simulink model "Cooperative_Localization_05_New2"  (R2016b)
settings: Solver=ode45  StartTime=0.0  StopTime=200  RelTol=1e-3  EnableMultiTasking=on
InitFcn:
  | Const_Coop_Local_05
undefined symbols (not defined in the file): alpha, AN, B, B_pseudo_inverse, BBT_inv, BN, D, Delta_form, Gama0, gamma0, gamma_0, gamma_1, H, K, k0_est, k1, k1_est, k2, KI, Ki_1, Ki_2, Ki_3, Ki_4, lambda, m_cont, Mb, Mu, n, N, n_cont, Observer_Gain, P_struct, Q, Q1, R, Rho1, Rho_0, rho_0, rho_1, t_cont, U_dot0_M
(part 2 of 3)

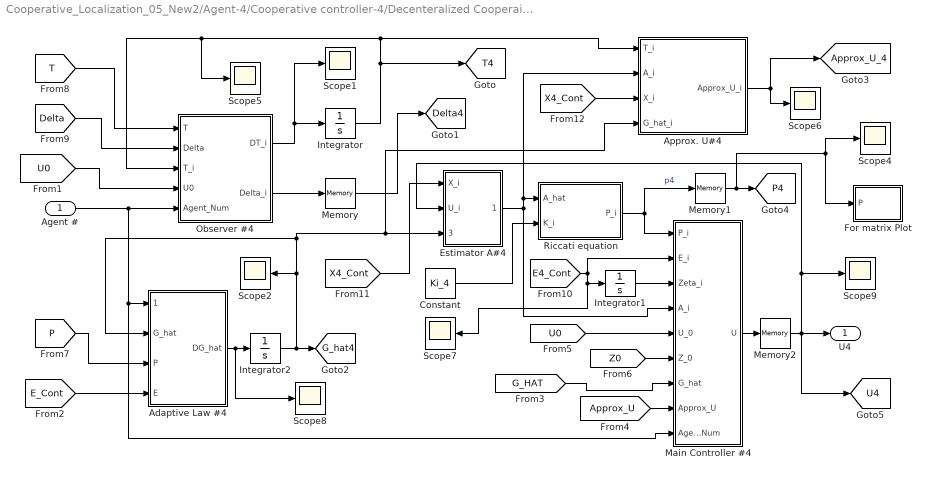
== system Cooperative_Localization_05_New2/Agent-4/Cooperative controller-4/Decenteralized Cooperaive Controller #4 ==
  Agent # : Inport
  Adaptive Law #4 : MATLAB Function  TreatAsAtomicUnit=on
  Approx. U#4 : MATLAB Function  TreatAsAtomicUnit=on
  Constant : Constant  Value=Ki_4
  Estimator A#4 : Subsystem
  For matrix Plot : Subsystem
  Integrator : Integrator  InitialCondition=zeros(n_cont,1)
  Integrator1 : Integrator  InitialCondition=zeros(n_cont,1)
  Integrator2 : Integrator  InitialCondition=zeros(t_cont,1)
  Main Controller #4 : MATLAB Function  TreatAsAtomicUnit=on
  Memory : Memory  X0=zeros(n_cont,1)
  Memory1 : Memory  X0=eye(n_cont)
  Memory2 : Memory  X0=zeros(m_cont,1)
  Observer #4 : MATLAB Function  TreatAsAtomicUnit=on
  Riccati equation : MATLAB Function  TreatAsAtomicUnit=on
  Scope{1..2,4..9} (8 alike) : Scope
  U4 : Outport
  tag scope: Approx_U_4=global, Delta4=global, G_hat4=global, P4=global, T4=global, U4=global
  wires:
  Memory/1 -> [Delta4]
  Agent #/1 -> Main Controller #4/9(Agent_Num), Adaptive Law #4/1(Agent_Num), Observer #4/5(Agent_Num)
  Observer #4/1(DT_i) -> Scope1/1, Integrator/1
  Observer #4/2(Delta_i) -> Memory/1
  [U0] -> Observer #4/4(U0)
  Adaptive Law #4/1(DG_hat) -> Scope8/1, Integrator2/1
  Integrator2/1 -> [G_hat4], Estimator A#4/3(G_hat_i), Approx. U#4/4(G_hat_i), Adaptive Law #4/2(G_hat), Scope2/1
  Integrator/1 -> Approx. U#4/1(T_i), Scope5/1, Observer #4/3(T_i), [T4]
  [Approx_U] -> Main Controller #4/8(Approx_U)
  [G_HAT] -> Main Controller #4/7(G_hat)
  [U0] -> Main Controller #4/5(U_0)
  [Z0] -> Main Controller #4/6(Z_0)
  Estimator A#4/1(A_hat_i) -> Main Controller #4/4(A_i), Riccati equation/1(A_hat), Approx. U#4/2(A_i)
  Riccati equation/1(P_i) -> Main Controller #4/1(P_i), Memory1/1  "p4"
  Main Controller #4/1(U) -> Memory2/1
  [P] -> Adaptive Law #4/3(P)
  [E_Cont] -> Adaptive Law #4/4(E)
  [T] -> Observer #4/1(T)
  [Delta] -> Observer #4/2(Delta)
  [E4_Cont] -> Main Controller #4/2(E_i), Integrator1/1, Scope7/1
  Integrator1/1 -> Main Controller #4/3(Zeta_i)
  [X4_Cont] -> Estimator A#4/1(X_i)
  [X4_Cont] -> Approx. U#4/3(X_i)
  Constant/1 -> Riccati equation/2(K_i)
  Memory2/1 -> [U4], Scope9/1, Estimator A#4/2(U_i), U4/1
  Memory1/1 -> For matrix Plot/1(P), Scope4/1, [P4]
  Approx. U#4/1(Approx_U_i) -> Scope6/1, [Approx_U_4]

== system Cooperative_Localization_05_New2/Agent-4/Relative positions-4/Differentiator_Scalar1 ==
  x_d : Inport
  Integrator : Integrator
  Integrator1 : Integrator
  Memory : Memory
  Scope : Scope
  Scope1 : Scope
  Sliding differentiator : MATLAB Function  TreatAsAtomicUnit=on
  Sliding differentiator1 : MATLAB Function  TreatAsAtomicUnit=on
  Sum : Sum  Inputs=|-+
  Dx_d : Outport
  wires:
  Memory/1 -> Dx_d/1
  Sliding differentiator1/1(Du1) -> Integrator/1
  Integrator/1 -> Sliding differentiator/1(u1)
  x_d/1 -> Sum/1
  Sum/1 -> Scope1/1, Sliding differentiator/2(e_inp), Sliding differentiator1/1(e_inp)
  Integrator1/1 -> Sum/2
  Sliding differentiator/1(u) -> Scope/1, Integrator1/1, Memory/1

== system Cooperative_Localization_05_New2/Agent-4/Relative positions-4/Differentiator_Scalar2 ==
  x_d : Inport
  Integrator : Integrator
  Integrator1 : Integrator
  Memory : Memory
  Scope : Scope
  Scope1 : Scope
  Sliding differentiator : MATLAB Function  TreatAsAtomicUnit=on
  Sliding differentiator1 : MATLAB Function  TreatAsAtomicUnit=on
  Sum : Sum  Inputs=|-+
  Dx_d : Outport
  wires:
  Sliding differentiator/1(u) -> Memory/1, Integrator1/1, Scope/1
  Integrator1/1 -> Sum/2
  Sum/1 -> Sliding differentiator1/1(e_inp), Sliding differentiator/2(e_inp), Scope1/1
  x_d/1 -> Sum/1
  Integrator/1 -> Sliding differentiator/1(u1)
  Sliding differentiator1/1(Du1) -> Integrator/1
  Memory/1 -> Dx_d/1

== system Cooperative_Localization_05_New2/Agent-4/Relative positions-4/Differentiator_Scalar3 ==
  x_d : Inport
  Integrator : Integrator
  Integrator1 : Integrator
  Memory : Memory
  Scope : Scope
  Scope1 : Scope
  Sliding differentiator : MATLAB Function  TreatAsAtomicUnit=on
  Sliding differentiator1 : MATLAB Function  TreatAsAtomicUnit=on
  Sum : Sum  Inputs=|-+
  Dx_d : Outport
  wires:
  Memory/1 -> Dx_d/1
  Sliding differentiator1/1(Du1) -> Integrator/1
  Integrator/1 -> Sliding differentiator/1(u1)
  x_d/1 -> Sum/1
  Sum/1 -> Scope1/1, Sliding differentiator/2(e_inp), Sliding differentiator1/1(e_inp)
  Integrator1/1 -> Sum/2
  Sliding differentiator/1(u) -> Scope/1, Integrator1/1, Memory/1

== system Cooperative_Localization_05_New2/Agent-4/Relative positions-4/Differentiator_Scalar4 ==
  x_d : Inport
  Integrator : Integrator
  Integrator1 : Integrator
  Memory : Memory
  Scope : Scope
  Scope1 : Scope
  Sliding differentiator : MATLAB Function  TreatAsAtomicUnit=on
  Sliding differentiator1 : MATLAB Function  TreatAsAtomicUnit=on
  Sum : Sum  Inputs=|-+
  Dx_d : Outport
  wires:
  Memory/1 -> Dx_d/1
  Sliding differentiator1/1(Du1) -> Integrator/1
  Integrator/1 -> Sliding differentiator/1(u1)
  x_d/1 -> Sum/1
  Sum/1 -> Scope1/1, Sliding differentiator/2(e_inp), Sliding differentiator1/1(e_inp)
  Integrator1/1 -> Sum/2
  Sliding differentiator/1(u) -> Scope/1, Integrator1/1, Memory/1

== system Cooperative_Localization_05_New2/Leader/Ali/Differentiator ==
  x_d : Inport
  Integrator : Integrator  InitialCondition=zeros(n_cont,1)
  Integrator1 : Integrator  InitialCondition=zeros(n_cont,1)
  Scope : Scope
  Scope1 : Scope
  Sliding differentiator : MATLAB Function  TreatAsAtomicUnit=on
  Sliding differentiator1 : MATLAB Function  TreatAsAtomicUnit=on
  Sum : Sum  Inputs=|-+
  Dx_d : Outport
  wires:
  Integrator1/1 -> Sum/2
  Sum/1 -> Sliding differentiator1/1(e), Sliding differentiator/2(e), Scope1/1
  x_d/1 -> Sum/1
  Integrator/1 -> Sliding differentiator/1(u1)
  Sliding differentiator1/1(Du1) -> Integrator/1
  Sliding differentiator/1(u) -> Dx_d/1, Integrator1/1, Scope/1

== system Cooperative_Localization_05_New2/Agent-1/Cooperative controller-1/Decenteralized Cooperaive Controller #1/Estimator A#1 ==
  X_i : Inport
  U_i : Inport  Port=2
  G_hat_i : Inport  Port=3
  Estimation Error : Subsystem
  For matrix Plot1 : Subsystem
  For matrix Plot2 : Subsystem
  Integrator : Integrator  InitialCondition=zeros(n_cont)
  Scope1 : Scope
  Scope5 : Scope
  parameter online identification : MATLAB Function  TreatAsAtomicUnit=on
  A_hat_i : Outport
  tag scope: A_hat1=global
  wires:
  parameter online identification/1(DA_hat) -> For matrix Plot2/1(A_dot), Scope5/1, Integrator/1
  Estimation Error/1(r) -> parameter online identification/1(r)
  Estimation Error/2(wt) -> parameter online identification/2(Wt)
  X_i/1 -> Estimation Error/1(X)
  U_i/1 -> Estimation Error/2(U)
  G_hat_i/1 -> Estimation Error/3(G_hat)
  Integrator/1 -> Scope1/1, For matrix Plot1/1(A), parameter online identification/3(A_hat), [A_hat1], A_hat_i/1

== system Cooperative_Localization_05_New2/Agent-1/Cooperative controller-1/Decenteralized Cooperaive Controller #1/For matrix Plot ==
  P : Inport
  MATLAB Function : MATLAB Function  TreatAsAtomicUnit=on
  To Workspace : ToWorkspace  VariableName=P_1_Cont  SaveFormat=Structure With Time  SampleTime=-1
  wires:
  P/1 -> MATLAB Function/1(u)
  MATLAB Function/1(y) -> To Workspace/1

== system Cooperative_Localization_05_New2/Agent-2/Cooperative controller-2/Decenteralized Cooperaive Controller #2/Estimator A#2 ==
  X_i : Inport
  U_i : Inport  Port=2
  G_hat_i : Inport  Port=3
  Estimation Error : Subsystem
  For matrix Plot1 : Subsystem
  For matrix Plot2 : Subsystem
  Integrator : Integrator  InitialCondition=zeros(n_cont)
  Scope1 : Scope
  Scope5 : Scope
  parameter online identification : MATLAB Function  TreatAsAtomicUnit=on
  A_hat_i : Outport
  tag scope: A_hat2=global
  wires:
  parameter online identification/1(DA_hat) -> For matrix Plot2/1(A_dot), Scope5/1, Integrator/1
  Estimation Error/1(r) -> parameter online identification/1(r)
  Estimation Error/2(wt) -> parameter online identification/2(Wt)
  X_i/1 -> Estimation Error/1(X)
  U_i/1 -> Estimation Error/2(U)
  G_hat_i/1 -> Estimation Error/3(G_hat)
  Integrator/1 -> Scope1/1, For matrix Plot1/1(A), parameter online identification/3(A_hat), [A_hat2], A_hat_i/1

== system Cooperative_Localization_05_New2/Agent-2/Cooperative controller-2/Decenteralized Cooperaive Controller #2/For matrix Plot ==
  P : Inport
  MATLAB Function : MATLAB Function  TreatAsAtomicUnit=on
  To Workspace : ToWorkspace  VariableName=P_2_Cont  SaveFormat=Structure With Time  SampleTime=-1
  wires:
  P/1 -> MATLAB Function/1(u)
  MATLAB Function/1(y) -> To Workspace/1

== system Cooperative_Localization_05_New2/Agent-3/Cooperative controller-3/Decenteralized Cooperaive Controller #3/Estimator A#3 ==
  X_i : Inport
  U_i : Inport  Port=2
  G_hat_i : Inport  Port=3
  Estimation Error : Subsystem
  For matrix Plot1 : Subsystem
  For matrix Plot2 : Subsystem
  Integrator : Integrator  InitialCondition=zeros(n_cont)
  Scope1 : Scope
  Scope5 : Scope
  parameter online identification : MATLAB Function  TreatAsAtomicUnit=on
  A_hat_i : Outport
  tag scope: A_hat3=global
  wires:
  parameter online identification/1(DA_hat) -> For matrix Plot2/1(A_dot), Scope5/1, Integrator/1
  Estimation Error/1(r) -> parameter online identification/1(r)
  Estimation Error/2(wt) -> parameter online identification/2(Wt)
  X_i/1 -> Estimation Error/1(X)
  U_i/1 -> Estimation Error/2(U)
  G_hat_i/1 -> Estimation Error/3(G_hat)
  Integrator/1 -> Scope1/1, For matrix Plot1/1(A), parameter online identification/3(A_hat), [A_hat3], A_hat_i/1

== system Cooperative_Localization_05_New2/Agent-3/Cooperative controller-3/Decenteralized Cooperaive Controller #3/For matrix Plot ==
  P : Inport
  MATLAB Function : MATLAB Function  TreatAsAtomicUnit=on
  To Workspace : ToWorkspace  VariableName=P_3_Cont  SaveFormat=Structure With Time  SampleTime=-1
  wires:
  P/1 -> MATLAB Function/1(u)
  MATLAB Function/1(y) -> To Workspace/1

== system Cooperative_Localization_05_New2/Agent-4/Cooperative controller-4/Decenteralized Cooperaive Controller #4/Estimator A#4 ==
  X_i : Inport
  U_i : Inport  Port=2
  G_hat_i : Inport  Port=3
  Estimation Error : Subsystem
  For matrix Plot1 : Subsystem
  For matrix Plot2 : Subsystem
  Integrator : Integrator  InitialCondition=zeros(n_cont)
  Scope1 : Scope
  Scope5 : Scope
  parameter online identification : MATLAB Function  TreatAsAtomicUnit=on
  A_hat_i : Outport
  tag scope: A_hat4=global
  wires:
  parameter online identification/1(DA_hat) -> For matrix Plot2/1(A_dot), Scope5/1, Integrator/1
  Estimation Error/1(r) -> parameter online identification/1(r)
  Estimation Error/2(wt) -> parameter online identification/2(Wt)
  X_i/1 -> Estimation Error/1(X)
  U_i/1 -> Estimation Error/2(U)
  G_hat_i/1 -> Estimation Error/3(G_hat)
  Integrator/1 -> Scope1/1, For matrix Plot1/1(A), parameter online identification/3(A_hat), [A_hat4], A_hat_i/1

== system Cooperative_Localization_05_New2/Agent-4/Cooperative controller-4/Decenteralized Cooperaive Controller #4/For matrix Plot ==
  P : Inport
  MATLAB Function : MATLAB Function  TreatAsAtomicUnit=on
  To Workspace : ToWorkspace  VariableName=P_4_Cont  SaveFormat=Structure With Time  SampleTime=-1
  wires:
  P/1 -> MATLAB Function/1(u)
  MATLAB Function/1(y) -> To Workspace/1

== system Cooperative_Localization_05_New2/Agent-1/Cooperative controller-1/Decenteralized Cooperaive Controller #1/Estimator A#1/Estimation Error ==
  X : Inport
  U : Inport  Port=2
  G_hat : Inport  Port=3
  Constant : Constant  Value=B
  Constant1 : Constant  Value=D
  Product : Product  Multiplication=Matrix(*)
  Product1 : Product  Multiplication=Matrix(*)
  Scope{1..5} (5 alike) : Scope
  Subsystem : Subsystem
  Subsystem1 : Subsystem
  Subsystem2 : Subsystem
  Subsystem3 : Subsystem
  Sum : Sum  Inputs=+--
  r : Outport
  wt : Outport  Port=2
  wires:
  G_hat/1 -> Product1/2
  Subsystem3/1(X_f) -> r/1, Scope4/1
  X/1 -> Subsystem/1(X), Subsystem3/1(X)
  Subsystem2/1(G_hatf) -> Sum/3, Scope2/1
  Subsystem1/1(Uf) -> Scope1/1, Sum/2
  Subsystem/1(Xf) -> Sum/1, Scope5/1
  Product1/1 -> Subsystem2/1(G_hat)
  Product/1 -> Subsystem1/1(U)
  Constant1/1 -> Product1/1
  U/1 -> Product/2
  Constant/1 -> Product/1
  Sum/1 -> wt/1, Scope3/1

== system Cooperative_Localization_05_New2/Agent-1/Cooperative controller-1/Decenteralized Cooperaive Controller #1/Estimator A#1/For matrix Plot1 ==
  A : Inport
  MATLAB Function : MATLAB Function  TreatAsAtomicUnit=on
  To Workspace : ToWorkspace  VariableName=A_hat_1  SaveFormat=Structure With Time  SampleTime=-1
  wires:
  MATLAB Function/1(y) -> To Workspace/1
  A/1 -> MATLAB Function/1(u)

== system Cooperative_Localization_05_New2/Agent-1/Cooperative controller-1/Decenteralized Cooperaive Controller #1/Estimator A#1/For matrix Plot2 ==
  A_dot : Inport
  MATLAB Function : MATLAB Function  TreatAsAtomicUnit=on
  To Workspace : ToWorkspace  VariableName=DA_hat_1  SaveFormat=Structure With Time  SampleTime=-1
  wires:
  A_dot/1 -> MATLAB Function/1(u)
  MATLAB Function/1(y) -> To Workspace/1

== system Cooperative_Localization_05_New2/Agent-2/Cooperative controller-2/Decenteralized Cooperaive Controller #2/Estimator A#2/Estimation Error ==
  X : Inport
  U : Inport  Port=2
  G_hat : Inport  Port=3
  Constant : Constant  Value=B
  Constant1 : Constant  Value=D
  Product : Product  Multiplication=Matrix(*)
  Product1 : Product  Multiplication=Matrix(*)
  Scope{1..5} (5 alike) : Scope
  Subsystem : Subsystem
  Subsystem1 : Subsystem
  Subsystem2 : Subsystem
  Subsystem3 : Subsystem
  Sum : Sum  Inputs=+--
  r : Outport
  wt : Outport  Port=2
  wires:
  G_hat/1 -> Product1/2
  Subsystem3/1(X_f) -> r/1, Scope4/1
  X/1 -> Subsystem/1(X), Subsystem3/1(X)
  Subsystem2/1(G_hatf) -> Sum/3, Scope2/1
  Subsystem1/1(Uf) -> Scope1/1, Sum/2
  Subsystem/1(Xf) -> Sum/1, Scope5/1
  Product1/1 -> Subsystem2/1(G_hat)
  Product/1 -> Subsystem1/1(U)
  Constant1/1 -> Product1/1
  U/1 -> Product/2
  Constant/1 -> Product/1
  Sum/1 -> wt/1, Scope3/1

== system Cooperative_Localization_05_New2/Agent-2/Cooperative controller-2/Decenteralized Cooperaive Controller #2/Estimator A#2/For matrix Plot1 ==
  A : Inport
  MATLAB Function : MATLAB Function  TreatAsAtomicUnit=on
  To Workspace : ToWorkspace  VariableName=A_hat_2  SaveFormat=Structure With Time  SampleTime=-1
  wires:
  MATLAB Function/1(y) -> To Workspace/1
  A/1 -> MATLAB Function/1(u)

== system Cooperative_Localization_05_New2/Agent-2/Cooperative controller-2/Decenteralized Cooperaive Controller #2/Estimator A#2/For matrix Plot2 ==
  A_dot : Inport
  MATLAB Function : MATLAB Function  TreatAsAtomicUnit=on
  To Workspace : ToWorkspace  VariableName=DA_hat_2  SaveFormat=Structure With Time  SampleTime=-1
  wires:
  A_dot/1 -> MATLAB Function/1(u)
  MATLAB Function/1(y) -> To Workspace/1

== system Cooperative_Localization_05_New2/Agent-3/Cooperative controller-3/Decenteralized Cooperaive Controller #3/Estimator A#3/Estimation Error ==
  X : Inport
  U : Inport  Port=2
  G_hat : Inport  Port=3
  Constant : Constant  Value=B
  Constant1 : Constant  Value=D
  Product : Product  Multiplication=Matrix(*)
  Product1 : Product  Multiplication=Matrix(*)
  Scope{1..5} (5 alike) : Scope
  Subsystem : Subsystem
  Subsystem1 : Subsystem
  Subsystem2 : Subsystem
  Subsystem3 : Subsystem
  Sum : Sum  Inputs=+--
  r : Outport
  wt : Outport  Port=2
  wires:
  G_hat/1 -> Product1/2
  Subsystem3/1(X_f) -> r/1, Scope4/1
  X/1 -> Subsystem/1(X), Subsystem3/1(X)
  Subsystem2/1(G_hatf) -> Sum/3, Scope2/1
  Subsystem1/1(Uf) -> Scope1/1, Sum/2
  Subsystem/1(Xf) -> Sum/1, Scope5/1
  Product1/1 -> Subsystem2/1(G_hat)
  Product/1 -> Subsystem1/1(U)
  Constant1/1 -> Product1/1
  U/1 -> Product/2
  Constant/1 -> Product/1
  Sum/1 -> wt/1, Scope3/1

== system Cooperative_Localization_05_New2/Agent-3/Cooperative controller-3/Decenteralized Cooperaive Controller #3/Estimator A#3/For matrix Plot1 ==
  A : Inport
  MATLAB Function : MATLAB Function  TreatAsAtomicUnit=on
  To Workspace : ToWorkspace  VariableName=A_hat_3  SaveFormat=Structure With Time  SampleTime=-1
  wires:
  MATLAB Function/1(y) -> To Workspace/1
  A/1 -> MATLAB Function/1(u)

== system Cooperative_Localization_05_New2/Agent-3/Cooperative controller-3/Decenteralized Cooperaive Controller #3/Estimator A#3/For matrix Plot2 ==
  A_dot : Inport
  MATLAB Function : MATLAB Function  TreatAsAtomicUnit=on
  To Workspace : ToWorkspace  VariableName=DA_hat_3  SaveFormat=Structure With Time  SampleTime=-1
  wires:
  A_dot/1 -> MATLAB Function/1(u)
  MATLAB Function/1(y) -> To Workspace/1

== system Cooperative_Localization_05_New2/Agent-4/Cooperative controller-4/Decenteralized Cooperaive Controller #4/Estimator A#4/Estimation Error ==
  X : Inport
  U : Inport  Port=2
  G_hat : Inport  Port=3
  Constant : Constant  Value=B
  Constant1 : Constant  Value=D
  Product : Product  Multiplication=Matrix(*)
  Product1 : Product  Multiplication=Matrix(*)
  Scope{1..5} (5 alike) : Scope
  Subsystem : Subsystem
  Subsystem1 : Subsystem
  Subsystem2 : Subsystem
  Subsystem3 : Subsystem
  Sum : Sum  Inputs=+--
  r : Outport
  wt : Outport  Port=2
  wires:
  G_hat/1 -> Product1/2
  Subsystem3/1(X_f) -> r/1, Scope4/1
  X/1 -> Subsystem/1(X), Subsystem3/1(X)
  Subsystem2/1(G_hatf) -> Sum/3, Scope2/1
  Subsystem1/1(Uf) -> Scope1/1, Sum/2
  Subsystem/1(Xf) -> Sum/1, Scope5/1
  Product1/1 -> Subsystem2/1(G_hat)
  Product/1 -> Subsystem1/1(U)
  Constant1/1 -> Product1/1
  U/1 -> Product/2
  Constant/1 -> Product/1
  Sum/1 -> wt/1, Scope3/1

== system Cooperative_Localization_05_New2/Agent-4/Cooperative controller-4/Decenteralized Cooperaive Controller #4/Estimator A#4/For matrix Plot1 ==
  A : Inport
  MATLAB Function : MATLAB Function  TreatAsAtomicUnit=on
  To Workspace : ToWorkspace  VariableName=A_hat_4  SaveFormat=Structure With Time  SampleTime=-1
  wires:
  MATLAB Function/1(y) -> To Workspace/1
  A/1 -> MATLAB Function/1(u)

== system Cooperative_Localization_05_New2/Agent-4/Cooperative controller-4/Decenteralized Cooperaive Controller #4/Estimator A#4/For matrix Plot2 ==
  A_dot : Inport
  MATLAB Function : MATLAB Function  TreatAsAtomicUnit=on
  To Workspace : ToWorkspace  VariableName=DA_hat_4  SaveFormat=Structure With Time  SampleTime=-1
  wires:
  A_dot/1 -> MATLAB Function/1(u)
  MATLAB Function/1(y) -> To Workspace/1

== system Cooperative_Localization_05_New2/Agent-1/Cooperative controller-1/Decenteralized Cooperaive Controller #1/Estimator A#1/Estimation Error/Subsystem ==
  X : Inport
  Demux : Demux
  Mux : Mux
  Transfer Fcn{,1..3} (4 alike) : TransferFcn  Numerator=[1 0]  Denominator=[1 1]
  Xf : Outport
  wires:
  Demux/1 -> Transfer Fcn/1
  Transfer Fcn/1 -> Mux/1
  Mux/1 -> Xf/1
  X/1 -> Demux/1
  Demux/2 -> Transfer Fcn1/1
  Transfer Fcn1/1 -> Mux/2
  Demux/3 -> Transfer Fcn2/1
  Transfer Fcn2/1 -> Mux/3
  Transfer Fcn3/1 -> Mux/4
  Demux/4 -> Transfer Fcn3/1

== system Cooperative_Localization_05_New2/Agent-1/Cooperative controller-1/Decenteralized Cooperaive Controller #1/Estimator A#1/Estimation Error/Subsystem1 ==
  U : Inport
  Demux : Demux
  Mux : Mux
  Transfer Fcn{1..4} (4 alike) : TransferFcn  Denominator=[1 1]
  Uf : Outport
  wires:
  U/1 -> Demux/1
  Mux/1 -> Uf/1
  Transfer Fcn1/1 -> Mux/1
  Demux/1 -> Transfer Fcn1/1
  Transfer Fcn2/1 -> Mux/2
  Demux/2 -> Transfer Fcn2/1
  Demux/3 -> Transfer Fcn3/1
  Transfer Fcn3/1 -> Mux/3
  Transfer Fcn4/1 -> Mux/4
  Demux/4 -> Transfer Fcn4/1

== system Cooperative_Localization_05_New2/Agent-1/Cooperative controller-1/Decenteralized Cooperaive Controller #1/Estimator A#1/Estimation Error/Subsystem2 ==
  G_hat : Inport
  Demux : Demux
  Mux : Mux
  Transfer Fcn{1..4} (4 alike) : TransferFcn  Denominator=[1 1]
  G_hatf : Outport
  wires:
  Demux/1 -> Transfer Fcn2/1
  Transfer Fcn2/1 -> Mux/1
  Mux/1 -> G_hatf/1
  G_hat/1 -> Demux/1
  Demux/2 -> Transfer Fcn1/1
  Transfer Fcn1/1 -> Mux/2
  Demux/3 -> Transfer Fcn3/1
  Transfer Fcn3/1 -> Mux/3
  Demux/4 -> Transfer Fcn4/1
  Transfer Fcn4/1 -> Mux/4

== system Cooperative_Localization_05_New2/Agent-1/Cooperative controller-1/Decenteralized Cooperaive Controller #1/Estimator A#1/Estimation Error/Subsystem3 ==
  X : Inport
  Demux : Demux
  Mux : Mux
  Transfer Fcn{1..4} (4 alike) : TransferFcn  Denominator=[1 1]
  X_f : Outport
  wires:
  X/1 -> Demux/1
  Mux/1 -> X_f/1
  Transfer Fcn2/1 -> Mux/1
  Demux/1 -> Transfer Fcn2/1
  Demux/2 -> Transfer Fcn1/1
  Transfer Fcn1/1 -> Mux/2
  Demux/3 -> Transfer Fcn3/1
  Transfer Fcn3/1 -> Mux/3
  Demux/4 -> Transfer Fcn4/1
  Transfer Fcn4/1 -> Mux/4

== system Cooperative_Localization_05_New2/Agent-2/Cooperative controller-2/Decenteralized Cooperaive Controller #2/Estimator A#2/Estimation Error/Subsystem ==
  X : Inport
  Demux : Demux
  Mux : Mux
  Transfer Fcn{,1..3} (4 alike) : TransferFcn  Numerator=[1 0]  Denominator=[1 1]
  Xf : Outport
  wires:
  Demux/1 -> Transfer Fcn/1
  Transfer Fcn/1 -> Mux/1
  Mux/1 -> Xf/1
  X/1 -> Demux/1
  Demux/2 -> Transfer Fcn1/1
  Transfer Fcn1/1 -> Mux/2
  Demux/3 -> Transfer Fcn2/1
  Transfer Fcn2/1 -> Mux/3
  Transfer Fcn3/1 -> Mux/4
  Demux/4 -> Transfer Fcn3/1

== system Cooperative_Localization_05_New2/Agent-2/Cooperative controller-2/Decenteralized Cooperaive Controller #2/Estimator A#2/Estimation Error/Subsystem1 ==
  U : Inport
  Demux : Demux
  Mux : Mux
  Transfer Fcn{1..4} (4 alike) : TransferFcn  Denominator=[1 1]
  Uf : Outport
  wires:
  U/1 -> Demux/1
  Mux/1 -> Uf/1
  Transfer Fcn1/1 -> Mux/1
  Demux/1 -> Transfer Fcn1/1
  Transfer Fcn2/1 -> Mux/2
  Demux/2 -> Transfer Fcn2/1
  Demux/3 -> Transfer Fcn3/1
  Transfer Fcn3/1 -> Mux/3
  Transfer Fcn4/1 -> Mux/4
  Demux/4 -> Transfer Fcn4/1

== system Cooperative_Localization_05_New2/Agent-2/Cooperative controller-2/Decenteralized Cooperaive Controller #2/Estimator A#2/Estimation Error/Subsystem2 ==
  G_hat : Inport
  Demux : Demux
  Mux : Mux
  Transfer Fcn{1..4} (4 alike) : TransferFcn  Denominator=[1 1]
  G_hatf : Outport
  wires:
  Demux/1 -> Transfer Fcn2/1
  Transfer Fcn2/1 -> Mux/1
  Mux/1 -> G_hatf/1
  G_hat/1 -> Demux/1
  Demux/2 -> Transfer Fcn1/1
  Transfer Fcn1/1 -> Mux/2
  Demux/3 -> Transfer Fcn3/1
  Transfer Fcn3/1 -> Mux/3
  Demux/4 -> Transfer Fcn4/1
  Transfer Fcn4/1 -> Mux/4

== system Cooperative_Localization_05_New2/Agent-2/Cooperative controller-2/Decenteralized Cooperaive Controller #2/Estimator A#2/Estimation Error/Subsystem3 ==
  X : Inport
  Demux : Demux
  Mux : Mux
  Transfer Fcn{1..4} (4 alike) : TransferFcn  Denominator=[1 1]
  X_f : Outport
  wires:
  X/1 -> Demux/1
  Mux/1 -> X_f/1
  Transfer Fcn2/1 -> Mux/1
  Demux/1 -> Transfer Fcn2/1
  Demux/2 -> Transfer Fcn1/1
  Transfer Fcn1/1 -> Mux/2
  Demux/3 -> Transfer Fcn3/1
  Transfer Fcn3/1 -> Mux/3
  Demux/4 -> Transfer Fcn4/1
  Transfer Fcn4/1 -> Mux/4

== system Cooperative_Localization_05_New2/Agent-3/Cooperative controller-3/Decenteralized Cooperaive Controller #3/Estimator A#3/Estimation Error/Subsystem ==
  X : Inport
  Demux : Demux
  Mux : Mux
  Transfer Fcn{,1..3} (4 alike) : TransferFcn  Numerator=[1 0]  Denominator=[1 1]
  Xf : Outport
  wires:
  Demux/1 -> Transfer Fcn/1
  Transfer Fcn/1 -> Mux/1
  Mux/1 -> Xf/1
  X/1 -> Demux/1
  Demux/2 -> Transfer Fcn1/1
  Transfer Fcn1/1 -> Mux/2
  Demux/3 -> Transfer Fcn2/1
  Transfer Fcn2/1 -> Mux/3
  Transfer Fcn3/1 -> Mux/4
  Demux/4 -> Transfer Fcn3/1

== system Cooperative_Localization_05_New2/Agent-3/Cooperative controller-3/Decenteralized Cooperaive Controller #3/Estimator A#3/Estimation Error/Subsystem1 ==
  U : Inport
  Demux : Demux
  Mux : Mux
  Transfer Fcn{1..4} (4 alike) : TransferFcn  Denominator=[1 1]
  Uf : Outport
  wires:
  U/1 -> Demux/1
  Mux/1 -> Uf/1
  Transfer Fcn1/1 -> Mux/1
  Demux/1 -> Transfer Fcn1/1
  Transfer Fcn2/1 -> Mux/2
  Demux/2 -> Transfer Fcn2/1
  Demux/3 -> Transfer Fcn3/1
  Transfer Fcn3/1 -> Mux/3
  Transfer Fcn4/1 -> Mux/4
  Demux/4 -> Transfer Fcn4/1

== system Cooperative_Localization_05_New2/Agent-3/Cooperative controller-3/Decenteralized Cooperaive Controller #3/Estimator A#3/Estimation Error/Subsystem2 ==
  G_hat : Inport
  Demux : Demux
  Mux : Mux
  Transfer Fcn{1..4} (4 alike) : TransferFcn  Denominator=[1 1]
  G_hatf : Outport
  wires:
  Demux/1 -> Transfer Fcn2/1
  Transfer Fcn2/1 -> Mux/1
  Mux/1 -> G_hatf/1
  G_hat/1 -> Demux/1
  Demux/2 -> Transfer Fcn1/1
  Transfer Fcn1/1 -> Mux/2
  Demux/3 -> Transfer Fcn3/1
  Transfer Fcn3/1 -> Mux/3
  Demux/4 -> Transfer Fcn4/1
  Transfer Fcn4/1 -> Mux/4

== system Cooperative_Localization_05_New2/Agent-3/Cooperative controller-3/Decenteralized Cooperaive Controller #3/Estimator A#3/Estimation Error/Subsystem3 ==
  X : Inport
  Demux : Demux
  Mux : Mux
  Transfer Fcn{1..4} (4 alike) : TransferFcn  Denominator=[1 1]
  X_f : Outport
  wires:
  X/1 -> Demux/1
  Mux/1 -> X_f/1
  Transfer Fcn2/1 -> Mux/1
  Demux/1 -> Transfer Fcn2/1
  Demux/2 -> Transfer Fcn1/1
  Transfer Fcn1/1 -> Mux/2
  Demux/3 -> Transfer Fcn3/1
  Transfer Fcn3/1 -> Mux/3
  Demux/4 -> Transfer Fcn4/1
  Transfer Fcn4/1 -> Mux/4

== system Cooperative_Localization_05_New2/Agent-4/Cooperative controller-4/Decenteralized Cooperaive Controller #4/Estimator A#4/Estimation Error/Subsystem ==
  X : Inport
  Demux : Demux
  Mux : Mux
  Transfer Fcn{,1..3} (4 alike) : TransferFcn  Numerator=[1 0]  Denominator=[1 1]
  Xf : Outport
  wires:
  Demux/1 -> Transfer Fcn/1
  Transfer Fcn/1 -> Mux/1
  Mux/1 -> Xf/1
  X/1 -> Demux/1
  Demux/2 -> Transfer Fcn1/1
  Transfer Fcn1/1 -> Mux/2
  Demux/3 -> Transfer Fcn2/1
  Transfer Fcn2/1 -> Mux/3
  Transfer Fcn3/1 -> Mux/4
  Demux/4 -> Transfer Fcn3/1

== system Cooperative_Localization_05_New2/Agent-4/Cooperative controller-4/Decenteralized Cooperaive Controller #4/Estimator A#4/Estimation Error/Subsystem1 ==
  U : Inport
  Demux : Demux
  Mux : Mux
  Transfer Fcn{1..4} (4 alike) : TransferFcn  Denominator=[1 1]
  Uf : Outport
  wires:
  U/1 -> Demux/1
  Mux/1 -> Uf/1
  Transfer Fcn1/1 -> Mux/1
  Demux/1 -> Transfer Fcn1/1
  Transfer Fcn2/1 -> Mux/2
  Demux/2 -> Transfer Fcn2/1
  Demux/3 -> Transfer Fcn3/1
  Transfer Fcn3/1 -> Mux/3
  Transfer Fcn4/1 -> Mux/4
  Demux/4 -> Transfer Fcn4/1

== system Cooperative_Localization_05_New2/Agent-4/Cooperative controller-4/Decenteralized Cooperaive Controller #4/Estimator A#4/Estimation Error/Subsystem2 ==
  G_hat : Inport
  Demux : Demux
  Mux : Mux
  Transfer Fcn{1..4} (4 alike) : TransferFcn  Denominator=[1 1]
  G_hatf : Outport
  wires:
  Demux/1 -> Transfer Fcn2/1
  Transfer Fcn2/1 -> Mux/1
  Mux/1 -> G_hatf/1
  G_hat/1 -> Demux/1
  Demux/2 -> Transfer Fcn1/1
  Transfer Fcn1/1 -> Mux/2
  Demux/3 -> Transfer Fcn3/1
  Transfer Fcn3/1 -> Mux/3
  Demux/4 -> Transfer Fcn4/1
  Transfer Fcn4/1 -> Mux/4

== system Cooperative_Localization_05_New2/Agent-4/Cooperative controller-4/Decenteralized Cooperaive Controller #4/Estimator A#4/Estimation Error/Subsystem3 ==
  X : Inport
  Demux : Demux
  Mux : Mux
  Transfer Fcn{1..4} (4 alike) : TransferFcn  Denominator=[1 1]
  X_f : Outport
  wires:
  X/1 -> Demux/1
  Mux/1 -> X_f/1
  Transfer Fcn2/1 -> Mux/1
  Demux/1 -> Transfer Fcn2/1
  Demux/2 -> Transfer Fcn1/1
  Transfer Fcn1/1 -> Mux/2
  Demux/3 -> Transfer Fcn3/1
  Transfer Fcn3/1 -> Mux/3
  Demux/4 -> Transfer Fcn4/1
  Transfer Fcn4/1 -> Mux/4

== matlab function Cooperative_Localization_05_New2/Agent-1/Cooperative controller-1/Choosing real control variables ==
  data: u output; U input
function u = fcn(U)

u = U(3:4);

end

== matlab function Cooperative_Localization_05_New2/Agent-1/Agent-1/MATLAB Function ==
  data: Px input; Py input; Vx input; out output; Vy input; Ax input; Ay input; t input
function out = fcn(Px,Py,Vx,Vy,Ax,Ay,t)

DPx = Vx;
DPy = Vy;

DVx = Ax - Vx * sin(0.2*t) + 0.5 * Px * cos(0.1*t);
DVy = Ay - Vy * sin(0.2*t) + 0.5 * Py * cos(0.1*t);

out = [DPx;DPy;DVx;DVy];

end

== matlab function Cooperative_Localization_05_New2/Agent-2/Agent-2/MATLAB Function ==
  data: Px input; Py input; Vx input; out output; Vy input; Ax input; Ay input; t input
function out = fcn(Px,Py,Vx,Vy,Ax,Ay,t)

DPx = Vx;
DPy = Vy;

DVx = Ax - Vx * sin(0.2*t) + 0.5 * Px * cos(0.1*t);
DVy = Ay - Vy * sin(0.2*t) + 0.5 * Py * cos(0.1*t);

out = [DPx;DPy;DVx;DVy];

end

== matlab function Cooperative_Localization_05_New2/Agent-2/Relative positions-2/Differentiator_Scalar1/Sliding differentiator ==
  data: u output; u1 input; e_inp input; k1 parameter
function u = fcn(u1,e_inp,k1)

b=k1;

if e_inp>0
    ABS = e_inp;
else
    ABS = -e_inp;
end

SGN = e_inp/(ABS + 0.01);

u = u1 - b*(ABS^0.5)*SGN;

end

== matlab function Cooperative_Localization_05_New2/Agent-2/Relative positions-2/Differentiator_Scalar1/Sliding differentiator1 ==
  data: Du1 output; e_inp input; k2 parameter
function Du1 = fcn(e_inp,k2)

a=k2;

if e_inp>0
    ABS = e_inp;
else
    ABS = -e_inp;
end
SGN = e_inp/(ABS + 0.01);

Du1 = - a*SGN;

end

== matlab function Cooperative_Localization_05_New2/Agent-2/Relative positions-2/Differentiator_Scalar2/Sliding differentiator ==
  data: u output; u1 input; e_inp input; k1 parameter
function u = fcn(u1,e_inp,k1)

b=k1;

if e_inp>0
    ABS = e_inp;
else
    ABS = -e_inp;
end

SGN = e_inp/(ABS + 0.01);

u = u1 - b*(ABS^0.5)*SGN;

end

== matlab function Cooperative_Localization_05_New2/Agent-2/Relative positions-2/Differentiator_Scalar2/Sliding differentiator1 ==
  data: Du1 output; e_inp input; k2 parameter
function Du1 = fcn(e_inp,k2)

a=k2;

if e_inp>0
    ABS = e_inp;
else
    ABS = -e_inp;
end
SGN = e_inp/(ABS + 0.01);

Du1 = - a*SGN;

end

== matlab function Cooperative_Localization_05_New2/Agent-1/observer-1 ==
  data: P_hat input; tau input; P0 input; P_rel_local input; P_rel0_local input; AN parameter; BN parameter; H parameter; DP_hat_local output; n parameter; N parameter; Num input; Mu parameter; Mb parameter; tau_i output; alpha parameter
function [DP_hat_local,tau_i] = fcn(P_hat,tau,P0,P_rel_local,P_rel0_local,AN,BN,H,n,N,Num,Mu,Mb,alpha)

P_hat_in = zeros(n,N);
P_rel_local_in = zeros(n,N);
tau_in = zeros(n,N);
for i=1:N
    P_hat_in(:,i) = P_hat((i-1)*n+1:(i*n),1); 
    P_rel_local_in(:,i) = P_rel_local((i-1)*n+1:(i*n),1); 
    tau_in(:,i) = tau((i-1)*n+1:(i*n),1);
end

e = BN(Num,Num)*(P_hat_in(:,Num) - (P0 + P_rel0_local));
Vec = zeros(n,1);
for i=1:N
    e = e + ( AN(Num,i)*(P_hat_in(:,Num) - (P_hat_in(:,i) + P_rel_local_in(:,i))) ); 
    Vec = Vec + ( H(Num,i)*tau_in(:,i) );    
end

SGN_vec = Vec./(abs(Vec)+alpha);
SGN = diag(SGN_vec);    

DP_hat_local = - ( Mu*e ) - ( SGN*Mb );
tau_i = e;

end

== matlab function Cooperative_Localization_05_New2/Agent-3/Relative positions-3/Differentiator_Scalar1/Sliding differentiator ==
  data: u output; u1 input; e_inp input; k1 parameter
function u = fcn(u1,e_inp,k1)

b=k1;

if e_inp>0
    ABS = e_inp;
else
    ABS = -e_inp;
end

SGN = e_inp/(ABS + 0.01);

u = u1 - b*(ABS^0.5)*SGN;

end

== matlab function Cooperative_Localization_05_New2/Agent-1/Relative positions-1/Differentiator_Scalar2/Sliding differentiator ==
  data: u output; u1 input; e_inp input; k1 parameter
function u = fcn(u1,e_inp,k1)

b=k1;

if e_inp>0
    ABS = e_inp;
else
    ABS = -e_inp;
end

SGN = e_inp/(ABS + 0.01);

u = u1 - b*(ABS^0.5)*SGN;

end

== matlab function Cooperative_Localization_05_New2/Agent-3/Relative positions-3/Differentiator_Scalar1/Sliding differentiator1 ==
  data: Du1 output; e_inp input; k2 parameter
function Du1 = fcn(e_inp,k2)

a=k2;

if e_inp>0
    ABS = e_inp;
else
    ABS = -e_inp;
end
SGN = e_inp/(ABS + 0.01);

Du1 = - a*SGN;

end

== matlab function Cooperative_Localization_05_New2/Agent-3/Relative positions-3/Differentiator_Scalar2/Sliding differentiator ==
  data: u output; u1 input; e_inp input; k1 parameter
function u = fcn(u1,e_inp,k1)

b=k1;

if e_inp>0
    ABS = e_inp;
else
    ABS = -e_inp;
end

SGN = e_inp/(ABS + 0.01);

u = u1 - b*(ABS^0.5)*SGN;

end

== matlab function Cooperative_Localization_05_New2/Agent-3/Relative positions-3/Differentiator_Scalar2/Sliding differentiator1 ==
  data: Du1 output; e_inp input; k2 parameter
function Du1 = fcn(e_inp,k2)

a=k2;

if e_inp>0
    ABS = e_inp;
else
    ABS = -e_inp;
end
SGN = e_inp/(ABS + 0.01);

Du1 = - a*SGN;

end

== matlab function Cooperative_Localization_05_New2/Agent-1/Cooperative controller-1/Decenteralized Cooperaive Controller #1/Adaptive Law #1 ==
  data: Agent_Num input; G_hat input; Gama0 parameter; P input; P_struct parameter; DG_hat output; E input; H parameter; D parameter; N parameter; n_cont parameter; t_cont parameter; Rho_0 parameter
function DG_hat = fcn(Agent_Num,G_hat,Gama0,P,P_struct,E,H,D,N,n_cont,t_cont,Rho_0)

P_struct(1).data = P.p1;
P_struct(2).data = P.p2;
P_struct(3).data = P.p3;
P_struct(4).data = P.p4;

Sum = zeros(t_cont,1);
for i=1:N  
    Sum = Sum + (H(i,Agent_Num) * D' * P_struct(i).data * E((i-1)*n_cont+1:(i*n_cont),1)); %Adaptive law
end

DG_hat = +( Gama0*Sum - (Rho_0*Gama0*G_hat) );
    
end

== matlab function Cooperative_Localization_05_New2/Agent-1/Relative positions-1/Differentiator_Scalar1/Sliding differentiator ==
  data: u output; u1 input; e_inp input; k1 parameter
function u = fcn(u1,e_inp,k1)

b=k1;

if e_inp>0
    ABS = e_inp;
else
    ABS = -e_inp;
end

SGN = e_inp/(ABS + 0.01);

u = u1 - b*(ABS^0.5)*SGN;

end

== matlab function Cooperative_Localization_05_New2/Agent-1/Relative positions-1/Differentiator_Scalar1/Sliding differentiator1 ==
  data: Du1 output; e_inp input; k2 parameter
function Du1 = fcn(e_inp,k2)

a=k2;

if e_inp>0
    ABS = e_inp;
else
    ABS = -e_inp;
end
SGN = e_inp/(ABS + 0.01);

Du1 = - a*SGN;

end

== matlab function Cooperative_Localization_05_New2/Agent-1/Relative positions-1/Differentiator_Scalar2/Sliding differentiator1 ==
  data: Du1 output; e_inp input; k2 parameter
function Du1 = fcn(e_inp,k2)

a=k2;

if e_inp>0
    ABS = e_inp;
else
    ABS = -e_inp;
end
SGN = e_inp/(ABS + 0.01);

Du1 = - a*SGN;

end

== matlab function Cooperative_Localization_05_New2/Agent-1/Relative positions-1/Differentiator_Scalar3/Sliding differentiator ==
  data: u output; u1 input; e_inp input; k1 parameter
function u = fcn(u1,e_inp,k1)

b=k1;

if e_inp>0
    ABS = e_inp;
else
    ABS = -e_inp;
end

SGN = e_inp/(ABS + 0.01);

u = u1 - b*(ABS^0.5)*SGN;

end

== matlab function Cooperative_Localization_05_New2/Agent-4/Relative positions-4/Differentiator_Scalar1/Sliding differentiator ==
  data: u output; u1 input; e_inp input; k1 parameter
function u = fcn(u1,e_inp,k1)

b=k1;

if e_inp>0
    ABS = e_inp;
else
    ABS = -e_inp;
end

SGN = e_inp/(ABS + 0.01);

u = u1 - b*(ABS^0.5)*SGN;

end

== matlab function Cooperative_Localization_05_New2/Agent-4/Relative positions-4/Differentiator_Scalar1/Sliding differentiator1 ==
  data: Du1 output; e_inp input; k2 parameter
function Du1 = fcn(e_inp,k2)

a=k2;

if e_inp>0
    ABS = e_inp;
else
    ABS = -e_inp;
end
SGN = e_inp/(ABS + 0.01);

Du1 = - a*SGN;

end

== matlab function Cooperative_Localization_05_New2/Agent-4/Relative positions-4/Differentiator_Scalar2/Sliding differentiator ==
  data: u output; u1 input; e_inp input; k1 parameter
function u = fcn(u1,e_inp,k1)

b=k1;

if e_inp>0
    ABS = e_inp;
else
    ABS = -e_inp;
end

SGN = e_inp/(ABS + 0.01);

u = u1 - b*(ABS^0.5)*SGN;

end

== matlab function Cooperative_Localization_05_New2/Agent-1/Relative positions-1/Differentiator_Scalar3/Sliding differentiator1 ==
  data: Du1 output; e_inp input; k2 parameter
function Du1 = fcn(e_inp,k2)

a=k2;

if e_inp>0
    ABS = e_inp;
else
    ABS = -e_inp;
end
SGN = e_inp/(ABS + 0.01);

Du1 = - a*SGN;

end

== matlab function Cooperative_Localization_05_New2/Agent-4/Relative positions-4/Differentiator_Scalar2/Sliding differentiator1 ==
  data: Du1 output; e_inp input; k2 parameter
function Du1 = fcn(e_inp,k2)

a=k2;

if e_inp>0
    ABS = e_inp;
else
    ABS = -e_inp;
end
SGN = e_inp/(ABS + 0.01);

Du1 = - a*SGN;

end

== matlab function Cooperative_Localization_05_New2/Agent-3/Agent-3/MATLAB Function ==
  data: Px input; Py input; Vx input; out output; Vy input; Ax input; Ay input; t input
function out = fcn(Px,Py,Vx,Vy,Ax,Ay,t)

DPx = Vx;
DPy = Vy;

DVx = Ax - Vx * sin(0.2*t) + 0.5 * Px * cos(0.1*t);
DVy = Ay - Vy * sin(0.2*t) + 0.5 * Py * cos(0.1*t);

out = [DPx;DPy;DVx;DVy];

end

== matlab function Cooperative_Localization_05_New2/Agent-4/Agent-4/MATLAB Function ==
  data: Px input; Py input; Vx input; out output; Vy input; Ax input; Ay input; t input
function out = fcn(Px,Py,Vx,Vy,Ax,Ay,t)

DPx = Vx;
DPy = Vy;

DVx = Ax - Vx * sin(0.2*t) + 0.5 * Px * cos(0.1*t);
DVy = Ay - Vy * sin(0.2*t) + 0.5 * Py * cos(0.1*t);

out = [DPx;DPy;DVx;DVy];

end

== matlab function Cooperative_Localization_05_New2/Agent-1/Relative positions-1/Differentiator_Scalar4/Sliding differentiator ==
  data: u output; u1 input; e_inp input; k1 parameter
function u = fcn(u1,e_inp,k1)

b=k1;

if e_inp>0
    ABS = e_inp;
else
    ABS = -e_inp;
end

SGN = e_inp/(ABS + 0.01);

u = u1 - b*(ABS^0.5)*SGN;

end

== matlab function Cooperative_Localization_05_New2/Leader/Agent-0/MATLAB Function ==
  data: Px input; Py input; Vx input; out output; Vy input; Ax input; Ay input; t input
function out = fcn(Px,Py,Vx,Vy,Ax,Ay,t)

DPx = Vx;
DPy = Vy;

DVx = Ax - Vx * sin(0.2*t) + 0.5 * Px * cos(0.1*t);
DVy = Ay - Vy * sin(0.2*t) + 0.5 * Py * cos(0.1*t);

out = [DPx;DPy;DVx;DVy];

end

== matlab function Cooperative_Localization_05_New2/Agent-2/Relative positions-2/Differentiator_Scalar3/Sliding differentiator ==
  data: u output; u1 input; e_inp input; k1 parameter
function u = fcn(u1,e_inp,k1)

b=k1;

if e_inp>0
    ABS = e_inp;
else
    ABS = -e_inp;
end

SGN = e_inp/(ABS + 0.01);

u = u1 - b*(ABS^0.5)*SGN;

end

== matlab function Cooperative_Localization_05_New2/Agent-2/Relative positions-2/Differentiator_Scalar3/Sliding differentiator1 ==
  data: Du1 output; e_inp input; k2 parameter
function Du1 = fcn(e_inp,k2)

a=k2;

if e_inp>0
    ABS = e_inp;
else
    ABS = -e_inp;
end
SGN = e_inp/(ABS + 0.01);

Du1 = - a*SGN;

end

== matlab function Cooperative_Localization_05_New2/Agent-1/Relative positions-1/Differentiator_Scalar4/Sliding differentiator1 ==
  data: Du1 output; e_inp input; k2 parameter
function Du1 = fcn(e_inp,k2)

a=k2;

if e_inp>0
    ABS = e_inp;
else
    ABS = -e_inp;
end
SGN = e_inp/(ABS + 0.01);

Du1 = - a*SGN;

end

== matlab function Cooperative_Localization_05_New2/Agent-2/Relative positions-2/Differentiator_Scalar4/Sliding differentiator ==
  data: u output; u1 input; e_inp input; k1 parameter
function u = fcn(u1,e_inp,k1)

b=k1;

if e_inp>0
    ABS = e_inp;
else
    ABS = -e_inp;
end

SGN = e_inp/(ABS + 0.01);

u = u1 - b*(ABS^0.5)*SGN;

end

== matlab function Cooperative_Localization_05_New2/Agent-2/Relative positions-2/Differentiator_Scalar4/Sliding differentiator1 ==
  data: Du1 output; e_inp input; k2 parameter
function Du1 = fcn(e_inp,k2)

a=k2;

if e_inp>0
    ABS = e_inp;
else
    ABS = -e_inp;
end
SGN = e_inp/(ABS + 0.01);

Du1 = - a*SGN;

end

== matlab function Cooperative_Localization_05_New2/Agent-2/Relative positions-2/Relative estimation ==
  data: V_rel input; d input; DP_est output; Dot_d input; P_est input; k0_est parameter; k1_est parameter
function DP_est = fcn(V_rel,d,Dot_d,P_est,k0_est,k1_est)

D = d*Dot_d;
e = (d^2) - (P_est'*P_est);
g = P_est'*V_rel;
DP_est = zeros(2,1);

if (V_rel'*V_rel) > 0
    beta = (k1_est*D + k0_est*e) / (k1_est*g+0.001);
    DP_est = beta * V_rel;
end

end

== matlab function Cooperative_Localization_05_New2/Agent-2/Relative positions-2/Relative estimation1 ==
  data: V_rel input; d input; DP_est output; Dot_d input; P_est input; k0_est parameter; k1_est parameter
function DP_est = fcn(V_rel,d,Dot_d,P_est,k0_est,k1_est)

D = d*Dot_d;
e = (d^2) - (P_est'*P_est);
g = P_est'*V_rel;
DP_est = zeros(2,1);

if (V_rel'*V_rel) > 0
    beta = (k1_est*D + k0_est*e) / (k1_est*g+0.001);
    DP_est = beta * V_rel;
end

end

== matlab function Cooperative_Localization_05_New2/Agent-2/Relative positions-2/Relative estimation2 ==
  data: V_rel input; d input; DP_est output; Dot_d input; P_est input; k0_est parameter; k1_est parameter
function DP_est = fcn(V_rel,d,Dot_d,P_est,k0_est,k1_est)

D = d*Dot_d;
e = (d^2) - (P_est'*P_est);
g = P_est'*V_rel;
DP_est = zeros(2,1);

if (V_rel'*V_rel) > 0
    beta = (k1_est*D + k0_est*e) / (k1_est*g+0.001);
    DP_est = beta * V_rel;
end

end

== matlab function Cooperative_Localization_05_New2/Agent-2/Relative positions-2/Relative estimation3 ==
  data: V_rel input; d input; DP_est output; Dot_d input; P_est input; k0_est parameter; k1_est parameter
function DP_est = fcn(V_rel,d,Dot_d,P_est,k0_est,k1_est)

D = d*Dot_d;
e = (d^2) - (P_est'*P_est);
g = P_est'*V_rel;
DP_est = zeros(2,1);

if (V_rel'*V_rel) > 0
    beta = (k1_est*D + k0_est*e) / (k1_est*g+0.001);
    DP_est = beta * V_rel;
end

end

== matlab function Cooperative_Localization_05_New2/Agent-2/Relative positions-2/Relative measurements ==
  data: P1 input; d output; P2 input
function d = fcn(P1,P2)

d = sqrt( (P2(1) - P1(1))^2 + (P2(2) - P1(2))^2 );

end

== matlab function Cooperative_Localization_05_New2/Agent-2/Relative positions-2/Relative measurements1 ==
  data: P1 input; d output; P2 input
function d = fcn(P1,P2)

d = sqrt( (P2(1) - P1(1))^2 + (P2(2) - P1(2))^2 );

end

== matlab function Cooperative_Localization_05_New2/Agent-2/Cooperative controller-2/Choosing real control variables ==
  data: u output; U input
function u = fcn(U)

u = U(3:4);

end

== matlab function Cooperative_Localization_05_New2/Agent-2/Cooperative controller-2/Decenteralized Cooperaive Controller #2/Adaptive Law #2 ==
  data: Agent_Num input; G_hat input; Gama0 parameter; P input; P_struct parameter; DG_hat output; E input; H parameter; D parameter; N parameter; n_cont parameter; t_cont parameter; Rho_0 parameter
function DG_hat = fcn(Agent_Num,G_hat,Gama0,P,P_struct,E,H,D,N,n_cont,t_cont,Rho_0)

P_struct(1).data = P.p1;
P_struct(2).data = P.p2;
P_struct(3).data = P.p3;
P_struct(4).data = P.p4;

Sum = zeros(t_cont,1);
for i=1:N  
    Sum = Sum + (H(i,Agent_Num) * D' * P_struct(i).data * E((i-1)*n_cont+1:(i*n_cont),1)); %Adaptive law
end

DG_hat = +( Gama0*Sum - (Rho_0*Gama0*G_hat) );
    
end

== matlab function Cooperative_Localization_05_New2/Agent-2/observer-1 ==
  data: P_hat input; tau input; P0 input; P_rel_local input; P_rel0_local input; AN parameter; BN parameter; H parameter; DP_hat_local output; n parameter; N parameter; Num input; Mu parameter; Mb parameter; tau_i output; alpha parameter
function [DP_hat_local,tau_i] = fcn(P_hat,tau,P0,P_rel_local,P_rel0_local,AN,BN,H,n,N,Num,Mu,Mb,alpha)

P_hat_in = zeros(n,N);
P_rel_local_in = zeros(n,N);
tau_in = zeros(n,N);
for i=1:N
    P_hat_in(:,i) = P_hat((i-1)*n+1:(i*n),1); 
    P_rel_local_in(:,i) = P_rel_local((i-1)*n+1:(i*n),1); 
    tau_in(:,i) = tau((i-1)*n+1:(i*n),1);
end

e = BN(Num,Num)*(P_hat_in(:,Num) - (P0 + P_rel0_local));
Vec = zeros(n,1);
for i=1:N
    e = e + ( AN(Num,i)*(P_hat_in(:,Num) - (P_hat_in(:,i) + P_rel_local_in(:,i))) ); 
    Vec = Vec + ( H(Num,i)*tau_in(:,i) );    
end

SGN_vec = Vec./(abs(Vec)+alpha);
SGN = diag(SGN_vec);    

DP_hat_local = - ( Mu*e ) - ( SGN*Mb );
tau_i = e;

end

== matlab function Cooperative_Localization_05_New2/Agent-2/Relative positions-2/Relative measurements2 ==
  data: P1 input; d output; P2 input
function d = fcn(P1,P2)

d = sqrt( (P2(1) - P1(1))^2 + (P2(2) - P1(2))^2 );

end

== matlab function Cooperative_Localization_05_New2/Agent-2/Relative positions-2/Relative measurements3 ==
  data: P1 input; d output; P2 input
function d = fcn(P1,P2)

d = sqrt( (P2(1) - P1(1))^2 + (P2(2) - P1(2))^2 );

end

== matlab function Cooperative_Localization_05_New2/Agent-1/Relative positions-1/Relative estimation ==
  data: V_rel input; d input; DP_est output; Dot_d input; P_est input; k0_est parameter; k1_est parameter
function DP_est = fcn(V_rel,d,Dot_d,P_est,k0_est,k1_est)

D = d*Dot_d;
e = (d^2) - (P_est'*P_est);
g = P_est'*V_rel;
DP_est = zeros(2,1);

if (V_rel'*V_rel) > 0
    beta = (k1_est*D + k0_est*e) / (k1_est*g+0.001);
    DP_est = beta * V_rel;
end

end

== matlab function Cooperative_Localization_05_New2/Agent-1/Relative positions-1/Relative estimation1 ==
  data: V_rel input; d input; DP_est output; Dot_d input; P_est input; k0_est parameter; k1_est parameter
function DP_est = fcn(V_rel,d,Dot_d,P_est,k0_est,k1_est)

D = d*Dot_d;
e = (d^2) - (P_est'*P_est);
g = P_est'*V_rel;
DP_est = zeros(2,1);

if (V_rel'*V_rel) > 0
    beta = (k1_est*D + k0_est*e) / (k1_est*g+0.001);
    DP_est = beta * V_rel;
end

end

== matlab function Cooperative_Localization_05_New2/Agent-1/Relative positions-1/Relative estimation2 ==
  data: V_rel input; d input; DP_est output; Dot_d input; P_est input; k0_est parameter; k1_est parameter
function DP_est = fcn(V_rel,d,Dot_d,P_est,k0_est,k1_est)

D = d*Dot_d;
e = (d^2) - (P_est'*P_est);
g = P_est'*V_rel;
DP_est = zeros(2,1);

if (V_rel'*V_rel) > 0
    beta = (k1_est*D + k0_est*e) / (k1_est*g+0.001);
    DP_est = beta * V_rel;
end

end

== matlab function Cooperative_Localization_05_New2/Agent-1/Relative positions-1/Relative estimation3 ==
  data: V_rel input; d input; DP_est output; Dot_d input; P_est input; k0_est parameter; k1_est parameter
function DP_est = fcn(V_rel,d,Dot_d,P_est,k0_est,k1_est)

D = d*Dot_d;
e = (d^2) - (P_est'*P_est);
g = P_est'*V_rel;
DP_est = zeros(2,1);

if (V_rel'*V_rel) > 0
    beta = (k1_est*D + k0_est*e) / (k1_est*g+0.001);
    DP_est = beta * V_rel;
end

end

== matlab function Cooperative_Localization_05_New2/Agent-1/Relative positions-1/Relative measurements ==
  data: P1 input; d output; P2 input
function d = fcn(P1,P2)

d = sqrt( (P2(1) - P1(1))^2 + (P2(2) - P1(2))^2 );

end

== matlab function Cooperative_Localization_05_New2/Agent-1/Relative positions-1/Relative measurements1 ==
  data: P1 input; d output; P2 input
function d = fcn(P1,P2)

d = sqrt( (P2(1) - P1(1))^2 + (P2(2) - P1(2))^2 );

end

== matlab function Cooperative_Localization_05_New2/Agent-1/Relative positions-1/Relative measurements2 ==
  data: P1 input; d output; P2 input
function d = fcn(P1,P2)

d = sqrt( (P2(1) - P1(1))^2 + (P2(2) - P1(2))^2 );

end

== matlab function Cooperative_Localization_05_New2/Agent-1/Relative positions-1/Relative measurements3 ==
  data: P1 input; d output; P2 input
function d = fcn(P1,P2)

d = sqrt( (P2(1) - P1(1))^2 + (P2(2) - P1(2))^2 );

end

== matlab function Cooperative_Localization_05_New2/Agent-3/Relative positions-3/Differentiator_Scalar3/Sliding differentiator ==
  data: u output; u1 input; e_inp input; k1 parameter
function u = fcn(u1,e_inp,k1)

b=k1;

if e_inp>0
    ABS = e_inp;
else
    ABS = -e_inp;
end

SGN = e_inp/(ABS + 0.01);

u = u1 - b*(ABS^0.5)*SGN;

end

== matlab function Cooperative_Localization_05_New2/Agent-3/Relative positions-3/Differentiator_Scalar3/Sliding differentiator1 ==
  data: Du1 output; e_inp input; k2 parameter
function Du1 = fcn(e_inp,k2)

a=k2;

if e_inp>0
    ABS = e_inp;
else
    ABS = -e_inp;
end
SGN = e_inp/(ABS + 0.01);

Du1 = - a*SGN;

end

== matlab function Cooperative_Localization_05_New2/Agent-3/Relative positions-3/Differentiator_Scalar4/Sliding differentiator ==
  data: u output; u1 input; e_inp input; k1 parameter
function u = fcn(u1,e_inp,k1)

b=k1;

if e_inp>0
    ABS = e_inp;
else
    ABS = -e_inp;
end

SGN = e_inp/(ABS + 0.01);

u = u1 - b*(ABS^0.5)*SGN;

end

== matlab function Cooperative_Localization_05_New2/Agent-3/Relative positions-3/Differentiator_Scalar4/Sliding differentiator1 ==
  data: Du1 output; e_inp input; k2 parameter
function Du1 = fcn(e_inp,k2)

a=k2;

if e_inp>0
    ABS = e_inp;
else
    ABS = -e_inp;
end
SGN = e_inp/(ABS + 0.01);

Du1 = - a*SGN;

end

== matlab function Cooperative_Localization_05_New2/Agent-3/Relative positions-3/Relative estimation ==
  data: V_rel input; d input; DP_est output; Dot_d input; P_est input; k0_est parameter; k1_est parameter
function DP_est = fcn(V_rel,d,Dot_d,P_est,k0_est,k1_est)

D = d*Dot_d;
e = (d^2) - (P_est'*P_est);
g = P_est'*V_rel;
DP_est = zeros(2,1);

if (V_rel'*V_rel) > 0
    beta = (k1_est*D + k0_est*e) / (k1_est*g+0.001);
    DP_est = beta * V_rel;
end

end

== matlab function Cooperative_Localization_05_New2/Agent-3/Relative positions-3/Relative estimation1 ==
  data: V_rel input; d input; DP_est output; Dot_d input; P_est input; k0_est parameter; k1_est parameter
function DP_est = fcn(V_rel,d,Dot_d,P_est,k0_est,k1_est)

D = d*Dot_d;
e = (d^2) - (P_est'*P_est);
g = P_est'*V_rel;
DP_est = zeros(2,1);

if (V_rel'*V_rel) > 0
    beta = (k1_est*D + k0_est*e) / (k1_est*g+0.001);
    DP_est = beta * V_rel;
end

end

== matlab function Cooperative_Localization_05_New2/Agent-3/Relative positions-3/Relative estimation2 ==
  data: V_rel input; d input; DP_est output; Dot_d input; P_est input; k0_est parameter; k1_est parameter
function DP_est = fcn(V_rel,d,Dot_d,P_est,k0_est,k1_est)

D = d*Dot_d;
e = (d^2) - (P_est'*P_est);
g = P_est'*V_rel;
DP_est = zeros(2,1);

if (V_rel'*V_rel) > 0
    beta = (k1_est*D + k0_est*e) / (k1_est*g+0.001);
    DP_est = beta * V_rel;
end

end

== matlab function Cooperative_Localization_05_New2/Agent-3/Cooperative controller-3/Choosing real control variables ==
  data: u output; U input
function u = fcn(U)

u = U(3:4);

end
